simulink subsystem "Controller"  (R2024b)
settings: Solver=VariableStepAuto  StartTime=0.0  StopTime=10.0  RelTol=1e-3
undefined symbols (not defined in the file or in its folder): flight_mode, Parameters, References
libraries: sharedtransform x13, eeGeneralControl x10, simulink x5, aerolibutil x2
(part 1 of 3)
settings Model: Creator=thesa  LastModifiedBy=thesa
settings RTWCC: GPUComputeCapability=3.5

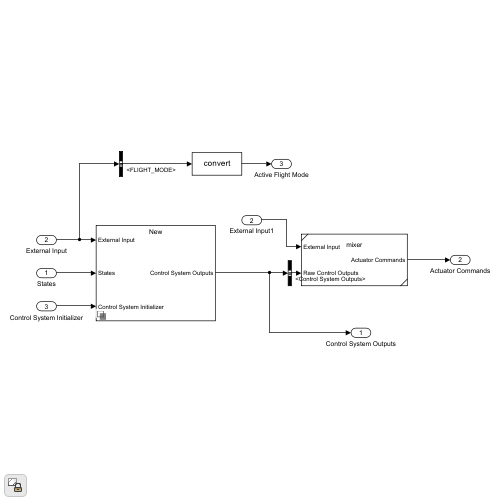
[thumbnail: Simulink's stored preview of the top-level diagram]
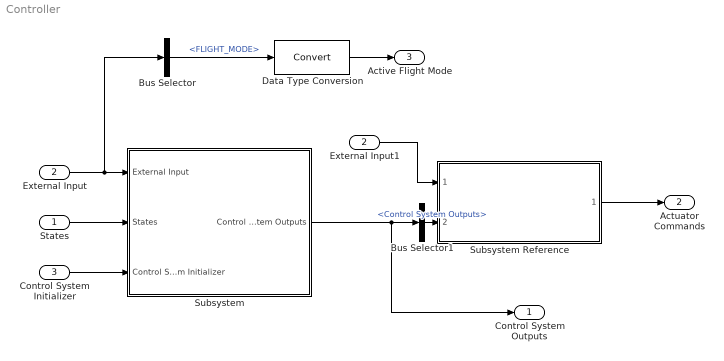
== system Controller ==
  States : Inport
  External Input : Inport  Port=2
  Control System Initializer : Inport  Port=3
  Bus Selector : BusSelector  OutputSignals=Pilot Input.FLIGHT_MODE
  Bus Selector1 : BusSelector  OutputSignals=Control System Outputs
  Data Type Conversion : DataTypeConversion  SaturateOnIntegerOverflow=off  RndMeth=Floor
  External Input1 : InportShadow  Port=2
  Subsystem : Subsystem  Variant=on  VariantControlMode=label  VariantControl=Choice  LabelModeActiveChoice=Choice_1
  Subsystem Reference : Subsystem  ReferencedSubsystem=mixer
  Control System Outputs : Outport
  Actuator Commands : Outport  Port=2
  Active Flight Mode : Outport  Port=3
  wires:
  Control System Initializer/1 -> Subsystem/3(Control System Initializer)
  States/1 -> Subsystem/2(States)
  External Input1/1 -> Subsystem Reference/1
  External Input/1 -> Bus Selector/1, Subsystem/1(External Input)
  Subsystem Reference/1 -> Actuator Commands/1
  Bus Selector/1 -> Data Type Conversion/1  "<FLIGHT_MODE>"
  Subsystem/1(Control System Outputs) -> Bus Selector1/1, Control System Outputs/1
  Data Type Conversion/1 -> Active Flight Mode/1
  Bus Selector1/1 -> Subsystem Reference/2  "<Control System Outputs>"

== system Controller/Subsystem ==
  External Input : Inport
  States : Inport  Port=2
  Control System Initializer : Inport  Port=3
  New : Subsystem  VariantControl=Choice_1
  OLD : Subsystem  VariantControl=Choice
  Control System Outputs : Outport

== system Controller/Subsystem/New ==
  External Input : Inport
  States : Inport  Port=2
  Control System Initializer : Inport  Port=3
  Bus Creator : BusCreator  Inputs=2
  External Input1 : InportShadow
  External Input2 : InportShadow
  Reference Source Selector Logic : Subsystem
  Rotational Motion Feedback Selector : Subsystem
  States2 : InportShadow  Port=2
  States3 : InportShadow  Port=2
  Translational Motion Feedback Selector : Subsystem
  Control System Outputs : Outport
  wires:
  Bus Creator/1 -> Control System Outputs/1
  Translational Motion Feedback Selector/2(Control System Outputs (intermediate)) -> Bus Creator/2  "Control System Outputs (intermediate)"
  Control System Initializer/1 -> Reference Source Selector Logic/3(Initialized Output (in))
  External Input/1 -> Reference Source Selector Logic/2(External Input)
  States/1 -> Reference Source Selector Logic/1(States)
  States3/1 -> Rotational Motion Feedback Selector/3(States)
  External Input2/1 -> Rotational Motion Feedback Selector/2(External Input)
  External Input1/1 -> Translational Motion Feedback Selector/2(External Input)
  States2/1 -> Translational Motion Feedback Selector/3(States)
  Translational Motion Feedback Selector/1(Initialized Output (out)) -> Rotational Motion Feedback Selector/1(Initialized Output (in))
  Rotational Motion Feedback Selector/1(Initialized Output (out)) -> Bus Creator/1  "Control System Outputs"
  Reference Source Selector Logic/1(Initialized Output (out)) -> Translational Motion Feedback Selector/1(Initialized Output (in))

== system Controller/Subsystem/OLD ==
  External Input : Inport
  States : Inport  Port=2
  Control System Initializer : Inport  Port=3
  Bus Selector : BusSelector  OutputSignals=Pilot Input.FLIGHT_MODE
  External Input1 : InportShadow
  Merge : Merge
  Switch Case : SwitchCase  CaseConditions={flight_mode.attitude_control}
  manual control (attitude only) : Subsystem  TreatAsAtomicUnit=on
  position_control + autonomous : Subsystem  TreatAsAtomicUnit=on
  Control System Outputs : Outport
  wires:
  Switch Case/2 -> position_control + autonomous/Action
  Bus Selector/1 -> Switch Case/1  "<FLIGHT_MODE>"
  position_control + autonomous/1(Control System Outputs) -> Merge/2
  States/1 -> manual control (attitude only)/2(States), position_control + autonomous/2(States)
  Switch Case/1 -> manual control (attitude only)/Action
  manual control (attitude only)/1(Control System Outputs) -> Merge/1
  External Input1/1 -> manual control (attitude only)/1(External Input), position_control + autonomous/1(External Input)
  Control System Initializer/1 -> manual control (attitude only)/3(Initialized Output), position_control + autonomous/3(Initialized Output)
  Merge/1 -> Control System Outputs/1
  External Input/1 -> Bus Selector/1

== system Controller/Subsystem/New/Reference Source Selector Logic ==
  States : Inport
  External Input : Inport  Port=2
  Initialized Output (in) : Inport  Port=3
  AUTONOMOUS : Subsystem
  External Input1 : InportShadow  Port=2
  External Input2 : InportShadow  Port=2
  External Input3 : InportShadow  Port=2
  Heading Reference Selection : Subsystem
  States1 : InportShadow
  States2 : InportShadow
  Thrust Reference Selection : Subsystem
  "[X, Y] and/or [Roll, Pitch] Reference Selection" : Subsystem
  Initialized Output (out) : Outport
  wires:
  External Input/1 -> Thrust Reference Selection/2(External Input)
  Initialized Output (in)/1 -> Thrust Reference Selection/1(Initialized Output (in))
  States/1 -> Heading Reference Selection/3(States)
  External Input1/1 -> Heading Reference Selection/2(External Input)
  External Input2/1 -> "[X, Y] and/or [Roll, Pitch] Reference Selection"/2(External Input)
  External Input3/1 -> AUTONOMOUS/2(External Input)
  States1/1 -> "[X, Y] and/or [Roll, Pitch] Reference Selection"/3(States)
  States2/1 -> AUTONOMOUS/3(States)
  AUTONOMOUS/1(Initialized Output (out)) -> Initialized Output (out)/1
  "[X, Y] and/or [Roll, Pitch] Reference Selection"/1(Initialized Output (out)) -> AUTONOMOUS/1(Initialized Output (in))
  Thrust Reference Selection/1(Initialized Output (out)) -> Heading Reference Selection/1(Initialized Output (in))
  Heading Reference Selection/1(Initialized Output (out)) -> "[X, Y] and/or [Roll, Pitch] Reference Selection"/1(Initialized Output (in))

== system Controller/Subsystem/New/Rotational Motion Feedback Selector ==
  Initialized Output (in) : Inport
  External Input : Inport  Port=2
  States : Inport  Port=3
  Bus Creator : BusCreator  Inputs=3
  Bus Selector1 : BusSelector  OutputSignals=External Input.Pilot Input.FLIGHT_MODE
  Merge : Merge
  Pass Through : Subsystem  TreatAsAtomicUnit=on
  Rate Transition : RateTransition  Commented=on  OutPortSampleTime=Parameters.Update_step_s.attitude
  Rate Transition1 : RateTransition  Commented=on
  Switch Case : SwitchCase  CaseConditions={[flight_mode.position_control, flight_mode.position_hold, flight_mode.autonomous, flight_mode.calibration, flight_mode.attitude_control]}
  Switch Case Action Subsystem : Subsystem  TreatAsAtomicUnit=on
  Initialized Output (out) : Outport
  wires:
  Bus Selector1/1 -> Switch Case/1  "<FLIGHT_MODE>"
  Switch Case Action Subsystem/1(Control System Outputs) -> Merge/2
  External Input/1 -> Bus Creator/2  "External Input"
  Pass Through/1(Control System Outputs) -> Merge/1
  Switch Case/2 -> Pass Through/Action
  Switch Case/1 -> Switch Case Action Subsystem/Action
  States/1 -> Bus Creator/3
  Initialized Output (in)/1 -> Bus Creator/1  "Control System Initializer"
  Merge/1 -> Initialized Output (out)/1
  Bus Creator/1 -> Pass Through/1(Combined Control Inputs), Switch Case Action Subsystem/1(Combined Control Inputs), Bus Selector1/1

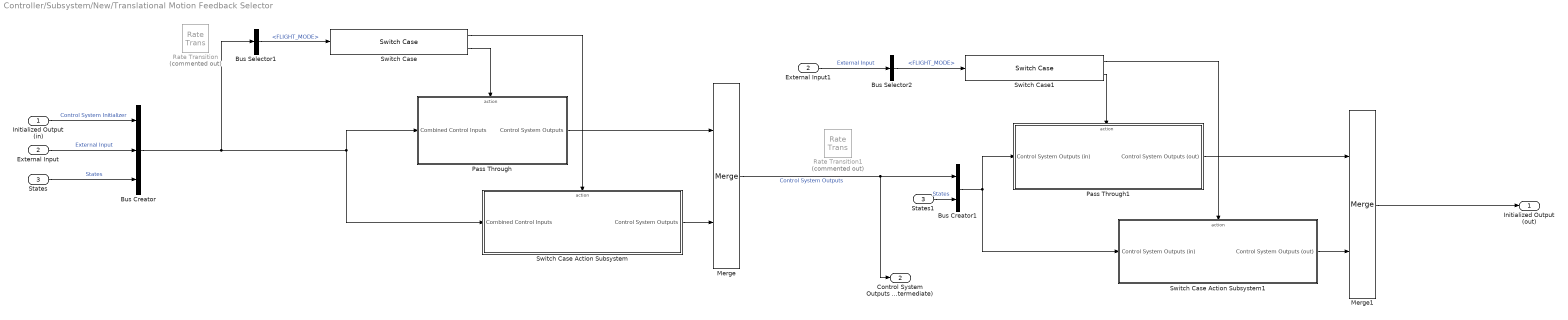
== system Controller/Subsystem/New/Translational Motion Feedback Selector ==
  Initialized Output (in) : Inport
  External Input : Inport  Port=2
  States : Inport  Port=3
  Bus Creator : BusCreator  Inputs=3
  Bus Creator1 : BusCreator  Inputs=2
  Bus Selector1 : BusSelector  OutputSignals=External Input.Pilot Input.FLIGHT_MODE
  Bus Selector2 : BusSelector  OutputSignals=Pilot Input.FLIGHT_MODE
  External Input1 : InportShadow  Port=2
  Merge : Merge
  Merge1 : Merge
  Pass Through : Subsystem  TreatAsAtomicUnit=on
  Pass Through1 : Subsystem  TreatAsAtomicUnit=on
  Rate Transition : RateTransition  Commented=on  OutPortSampleTime=Parameters.Update_step_s.position
  Rate Transition1 : RateTransition  Commented=on  Integrity=off  Deterministic=off
  States1 : InportShadow  Port=3
  Switch Case : SwitchCase  CaseConditions={[flight_mode.position_control, flight_mode.position_hold, flight_mode.autonomous]}
  Switch Case Action Subsystem : Subsystem  TreatAsAtomicUnit=on
  Switch Case Action Subsystem1 : Subsystem  TreatAsAtomicUnit=on
  Switch Case1 : SwitchCase  CaseConditions={[flight_mode.position_control, flight_mode.position_hold, flight_mode.autonomous]}
  Initialized Output (out) : Outport
  Control System Outputs (intermediate) : Outport  Port=2
  wires:
  Bus Selector1/1 -> Switch Case/1  "<FLIGHT_MODE>"
  Switch Case Action Subsystem/1(Control System Outputs) -> Merge/2
  Pass Through/1(Control System Outputs) -> Merge/1
  Switch Case/2 -> Pass Through/Action
  Switch Case/1 -> Switch Case Action Subsystem/Action
  Initialized Output (in)/1 -> Bus Creator/1  "Control System Initializer"
  States/1 -> Bus Creator/3  "States"
  External Input/1 -> Bus Creator/2  "External Input"
  Pass Through1/1(Control System Outputs (out)) -> Merge1/1
  Switch Case1/2 -> Pass Through1/Action
  Bus Creator1/1 -> Pass Through1/1(Control System Outputs (in)), Switch Case Action Subsystem1/1(Control System Outputs (in))
  Switch Case Action Subsystem1/1(Control System Outputs (out)) -> Merge1/2
  Bus Selector2/1 -> Switch Case1/1  "<FLIGHT_MODE>"
  Switch Case1/1 -> Switch Case Action Subsystem1/Action
  External Input1/1 -> Bus Selector2/1  "External Input"
  States1/1 -> Bus Creator1/2  "States"
  Merge1/1 -> Initialized Output (out)/1
  Merge/1 -> Bus Creator1/1, Control System Outputs (intermediate)/1  "Control System Outputs"
  Bus Creator/1 -> Bus Selector1/1, Pass Through/1(Combined Control Inputs), Switch Case Action Subsystem/1(Combined Control Inputs)

== system Controller/Subsystem/OLD/manual control (attitude only) ==
  External Input : Inport
  States : Inport  Port=2
  Initialized Output : Inport  Port=3
  Action Port : ActionPort  InitializeStates=reset
  Subsystem : Subsystem
  Control System Outputs : Outport
  wires:
  Initialized Output/1 -> Subsystem/3(Initialized Output)
  States/1 -> Subsystem/2(States)
  External Input/1 -> Subsystem/1(External Input)
  Subsystem/1(Control Outputs) -> Control System Outputs/1

== system Controller/Subsystem/OLD/position_control + autonomous ==
  External Input : Inport
  States : Inport  Port=2
  Initialized Output : Inport  Port=3
  Action Port : ActionPort  InitializeStates=reset
  Bus Selector : BusSelector  OutputSignals=Control Gains.K_matrix_control.EN
  Guidance : Subsystem
  If : If  IfExpression=u1
  If Action Subsystem : Subsystem  TreatAsAtomicUnit=on
  K-matrix control : Subsystem  TreatAsAtomicUnit=on
  Merge : Merge
  Control System Outputs : Outport
  wires:
  Initialized Output/1 -> Guidance/3(Initialized Output)
  Merge/1 -> Control System Outputs/1
  External Input/1 -> Bus Selector/1, K-matrix control/2(External Inputs), If Action Subsystem/2(External Inputs), Guidance/1(external_input)
  States/1 -> If Action Subsystem/3(States), K-matrix control/3(States), Guidance/2(States)
  Guidance/1(Initialized Output (with references)) -> If Action Subsystem/1(Initialized Output (with references)), K-matrix control/1(Initialized Output (with references))
  If/2 -> If Action Subsystem/Action
  If Action Subsystem/1(Control System Outputs) -> Merge/2
  If/1 -> K-matrix control/Action
  K-matrix control/1(Control System Outputs) -> Merge/1
  Bus Selector/1 -> If/1  "<EN>"

== system Controller/Subsystem/New/Reference Source Selector Logic/AUTONOMOUS ==
  Initialized Output (in) : Inport
  External Input : Inport  Port=2
  States : Inport  Port=3
  Bus Selector : BusSelector  OutputSignals=Pilot Input.FLIGHT_MODE
  External Input1 : InportShadow  Port=2
  Initialized Output (in)1 : InportShadow
  Merge : Merge
  Pass Through : Subsystem  TreatAsAtomicUnit=on
  Switch Case : SwitchCase  CaseConditions={flight_mode.autonomous}
  Use minimum-snap trajectory solution : Subsystem  TreatAsAtomicUnit=on
  Initialized Output (out) : Outport
  wires:
  Initialized Output (in)/1 -> Use minimum-snap trajectory solution/3(Initialized Output)
  States/1 -> Use minimum-snap trajectory solution/2(States)
  Switch Case/1 -> Use minimum-snap trajectory solution/Action
  Bus Selector/1 -> Switch Case/1  "<FLIGHT_MODE>"
  Merge/1 -> Initialized Output (out)/1
  External Input/1 -> Bus Selector/1
  Initialized Output (in)1/1 -> Pass Through/1(Initialized Output (in))
  Use minimum-snap trajectory solution/1(Modified-Initialized Output) -> Merge/2
  External Input1/1 -> Use minimum-snap trajectory solution/1(External Input)
  Switch Case/2 -> Pass Through/Action
  Pass Through/1(Initialized Output (out)) -> Merge/1

== system Controller/Subsystem/New/Reference Source Selector Logic/Heading Reference Selection ==
  Initialized Output (in) : Inport
  External Input : Inport  Port=2
  States : Inport  Port=3
  Bus Selector : BusSelector  OutputSignals=Pilot Input.FLIGHT_MODE
  Direct Yaw Command : Subsystem  TreatAsAtomicUnit=on
  External Input1 : InportShadow  Port=2
  Initialized Output (in)1 : InportShadow
  Merge : Merge
  Pass Through : Subsystem  TreatAsAtomicUnit=on
  Switch Case : SwitchCase  CaseConditions={[flight_mode.position_control, flight_mode.position_hold, flight_mode.calibration, flight_mode.attitude_control]}
  Initialized Output (out) : Outport
  wires:
  Initialized Output (in)1/1 -> Direct Yaw Command/1(Initialized Output (in))
  Merge/1 -> Initialized Output (out)/1
  Switch Case/2 -> Pass Through/Action
  Switch Case/1 -> Direct Yaw Command/Action
  Pass Through/1(Initialized Output (out)) -> Merge/1
  Initialized Output (in)/1 -> Pass Through/1(Initialized Output (in))
  Direct Yaw Command/1(Initialized Output (out)) -> Merge/2
  States/1 -> Direct Yaw Command/3(States)
  Bus Selector/1 -> Switch Case/1  "<FLIGHT_MODE>"
  External Input1/1 -> Direct Yaw Command/2(External Input)
  External Input/1 -> Bus Selector/1

== system Controller/Subsystem/New/Reference Source Selector Logic/Thrust Reference Selection ==
  Initialized Output (in) : Inport
  External Input : Inport  Port=2
  Bus Selector : BusSelector  OutputSignals=Pilot Input.FLIGHT_MODE
  Direct Thrust Command : Subsystem  TreatAsAtomicUnit=on
  Direct Z Position Command : Subsystem  TreatAsAtomicUnit=on
  External Input1 : InportShadow  Port=2
  External Input2 : InportShadow  Port=2
  Initialized Output (in)1 : InportShadow
  Initialized Output (in)2 : InportShadow
  Merge : Merge  Inputs=3
  Pass Through : Subsystem  TreatAsAtomicUnit=on
  Switch Case : SwitchCase  CaseConditions={[flight_mode.position_control, flight_mode.position_hold], [flight_mode.calibration, flight_mode.attitude_control]}
  Initialized Output (out) : Outport
  wires:
  Switch Case/1 -> Direct Z Position Command/Action
  Switch Case/3 -> Pass Through/Action
  Bus Selector/1 -> Switch Case/1  "<FLIGHT_MODE>"
  Switch Case/2 -> Direct Thrust Command/Action
  Pass Through/1(Initialized Output (out)) -> Merge/1
  Direct Z Position Command/1(Initialized Output (out)) -> Merge/3
  Direct Thrust Command/1(Initialized Output (out)) -> Merge/2
  Merge/1 -> Initialized Output (out)/1
  Initialized Output (in)/1 -> Pass Through/1(Initialized Output (in))
  Initialized Output (in)1/1 -> Direct Thrust Command/1(Initialized Output (in))
  Initialized Output (in)2/1 -> Direct Z Position Command/1(Initialized Output (in))
  External Input/1 -> Bus Selector/1
  External Input1/1 -> Direct Z Position Command/2(External Input)
  External Input2/1 -> Direct Thrust Command/2(External Input)

== system Controller/Subsystem/New/Reference Source Selector Logic/[X, Y] and//or [Roll, Pitch] Reference Selection ==
  Initialized Output (in) : Inport
  External Input : Inport  Port=2
  States : Inport  Port=3
  Bus Selector : BusSelector  OutputSignals=Pilot Input.FLIGHT_MODE
  Direct Roll and Pitch Command : Subsystem  TreatAsAtomicUnit=on
  "Direct XY Position Command " : Subsystem  TreatAsAtomicUnit=on
  External Input1 : InportShadow  Port=2
  External Input2 : InportShadow  Port=2
  Initialized Output (in)1 : InportShadow
  Initialized Output (in)2 : InportShadow
  Merge : Merge  Inputs=3
  Pass Through : Subsystem  TreatAsAtomicUnit=on
  Switch Case : SwitchCase  CaseConditions={[flight_mode.position_control, flight_mode.position_hold], [flight_mode.calibration, flight_mode.attitude_control]}
  Initialized Output (out) : Outport
  wires:
  Initialized Output (in)1/1 -> Direct Roll and Pitch Command/1(Initialized Output (in))
  Merge/1 -> Initialized Output (out)/1
  Switch Case/3 -> Pass Through/Action
  Switch Case/2 -> Direct Roll and Pitch Command/Action
  Pass Through/1(Initialized Output (out)) -> Merge/1
  Initialized Output (in)/1 -> Pass Through/1(Initialized Output (in))
  Direct Roll and Pitch Command/1(Initialized Output (out)) -> Merge/2
  States/1 -> "Direct XY Position Command "/3(States)
  External Input1/1 -> Direct Roll and Pitch Command/2(External Input)
  Switch Case/1 -> "Direct XY Position Command "/Action
  "Direct XY Position Command "/1(Initialized Output (out)) -> Merge/3
  Initialized Output (in)2/1 -> "Direct XY Position Command "/1(Initialized Output (in))
  External Input2/1 -> "Direct XY Position Command "/2(External Input)
  External Input/1 -> Bus Selector/1
  Bus Selector/1 -> Switch Case/1  "<FLIGHT_MODE>"

== system Controller/Subsystem/New/Rotational Motion Feedback Selector/Pass Through ==
  Combined Control Inputs : Inport
  Action Port : ActionPort  InitializeStates=reset
  Bus Selector : BusSelector  OutputSignals=Control System Initializer
  Control System Outputs : Outport
  wires:
  Bus Selector/1 -> Control System Outputs/1  "<Control System Initializer>"
  Combined Control Inputs/1 -> Bus Selector/1

== system Controller/Subsystem/New/Rotational Motion Feedback Selector/Switch Case Action Subsystem ==
  Combined Control Inputs : Inport
  Action Port : ActionPort  InitializeStates=reset
  Add : Sum  Inputs=++|
  Attitude Control : Subsystem  ReferencedSubsystem=Attitude_Control
  Bus Assignment : BusAssignment  AssignedSignals=Control Outputs.Tau
  Bus Selector : BusSelector  OutputSignals=Control System Initializer.References.reconstructed.q,Control System Initializer.References.reconstructed.omega,Control System Initializer.References.reconstructed.omega_dot,States,External Input
  Bus Selector1 : BusSelector  OutputSignals=Control System Initializer,Control System Initializer.References.reconstructed.Tau
  Combined Control Inputs1 : InportShadow
  Terminator : Terminator
  Control System Outputs : Outport
  wires:
  Bus Selector/1 -> Attitude Control/1  "<q>"
  Bus Selector/2 -> Attitude Control/2  "<omega>"
  Bus Selector/3 -> Attitude Control/3  "<omega_dot>"
  Bus Selector/4 -> Attitude Control/4  "<States>"
  Bus Selector/5 -> Attitude Control/5  "<External Input>"
  Bus Selector1/2 -> Add/1  "<Tau>"
  Add/1 -> Bus Assignment/2
  Combined Control Inputs/1 -> Bus Selector/1
  Bus Assignment/1 -> Control System Outputs/1
  Combined Control Inputs1/1 -> Bus Selector1/1
  Attitude Control/1 -> Add/2
  Bus Selector1/1 -> Bus Assignment/1  "<Control System Initializer>"
  Attitude Control/2 -> Terminator/1

== system Controller/Subsystem/New/Translational Motion Feedback Selector/Pass Through ==
  Combined Control Inputs : Inport
  Action Port : ActionPort  InitializeStates=reset
  Bus Creator : BusCreator  Inputs=2
  Bus Selector : BusSelector  OutputSignals=Control System Initializer
  Constant : Constant  Value=zeros(3,1)
  Reshape : Reshape
  Control System Outputs : Outport
  wires:
  Bus Selector/1 -> Bus Creator/1  "<Control System Initializer>"
  Combined Control Inputs/1 -> Bus Selector/1
  Bus Creator/1 -> Control System Outputs/1  "Control System Outputs"
  Constant/1 -> Reshape/1
  Reshape/1 -> Bus Creator/2  "thrust_ref"

== system Controller/Subsystem/New/Translational Motion Feedback Selector/Pass Through1 ==
  Control System Outputs (in) : Inport
  Action Port : ActionPort  InitializeStates=reset
  Bus Selector : BusSelector  OutputSignals=Control System Outputs.Control System Initializer
  Control System Outputs (out) : Outport
  wires:
  Bus Selector/1 -> Control System Outputs (out)/1  "<Control System Initializer>"
  Control System Outputs (in)/1 -> Bus Selector/1

== system Controller/Subsystem/New/Translational Motion Feedback Selector/Switch Case Action Subsystem ==
  Combined Control Inputs : Inport
  Action Port : ActionPort  InitializeStates=reset
  Bus Selector : BusSelector  OutputSignals=Control System Initializer,External Input,States
  Translational Motion Control : Subsystem  VariantControl=Choice_1
  Control System Outputs : Outport
  wires:
  Bus Selector/2 -> Translational Motion Control/2(External Inputs)  "<External Input>"
  Combined Control Inputs/1 -> Bus Selector/1
  Bus Selector/3 -> Translational Motion Control/3(States)  "<States>"
  Bus Selector/1 -> Translational Motion Control/1(Initialized Output (with references))  "<Control System Initializer>"
  Translational Motion Control/1(Control System Outputs) -> Control System Outputs/1

== system Controller/Subsystem/New/Translational Motion Feedback Selector/Switch Case Action Subsystem1 ==
  Control System Outputs (in) : Inport
  Action Port : ActionPort  InitializeStates=reset
  Bus Selector : BusSelector  OutputSignals=Control System Outputs.thrust_ref,Control System Outputs
  Translational Motion Control : Subsystem  VariantControl=Choice_1
  Control System Outputs (out) : Outport
  wires:
  Control System Outputs (in)/1 -> Bus Selector/1
  Bus Selector/2 -> Translational Motion Control/2(Control System Outputs (in))  "<Control System Outputs>"
  Translational Motion Control/1(Control System Outputs (out)) -> Control System Outputs (out)/1
  Bus Selector/1 -> Translational Motion Control/1(thrust_ref)  "<thrust_ref>"

== system Controller/Subsystem/OLD/manual control (attitude only)/Subsystem ==
  External Input : Inport
  States : Inport  Port=2
  Initialized Output : Inport  Port=3
  External Input1 : InportShadow
  Map User Input : Subsystem
  Reshape2 : Reshape  OutputDimensionality=Column vector (2-D)
  States1 : InportShadow  Port=2
  Subsystem : Subsystem
  Subsystem1 : Subsystem
  Subsystem2 : Subsystem  Commented=on
  Control Outputs : Outport
  wires:
  Initialized Output/1 -> Subsystem1/6(Initialized Output)
  States/1 -> Map User Input/2(States)
  Subsystem1/1(Control Outputs) -> Control Outputs/1
  External Input/1 -> Map User Input/1(External Input)
  Map User Input/2(att_ref) -> Subsystem/1(att_ref), Subsystem1/2(att_ref)
  Reshape2/1 -> Subsystem/2(omega_ref), Subsystem1/3(omega_ref)
  Map User Input/1(T_ref) -> Subsystem1/1(T)  "T"
  Map User Input/3(omega_ref) -> Reshape2/1
  Map User Input/4(omega_dot_ref) -> Subsystem/3(omega_dot_ref)
  External Input1/1 -> Subsystem/5(External Input)
  States1/1 -> Subsystem/4(States)
  Subsystem/2(Tau) -> Subsystem1/5(Tau)
  Subsystem/1(omega_dot) -> Subsystem1/4(omega_dot)

== system Controller/Subsystem/OLD/position_control + autonomous/Guidance ==
  external_input : Inport
  States : Inport  Port=2
  Initialized Output : Inport  Port=3
  Trajectory Solution Evaluator : Subsystem
  Initialized Output (with references) : Outport
  wires:
  Initialized Output/1 -> Trajectory Solution Evaluator/3(Initialized Output)
  States/1 -> Trajectory Solution Evaluator/2(States)
  Trajectory Solution Evaluator/1(Initialized Output (with references)) -> Initialized Output (with references)/1
  external_input/1 -> Trajectory Solution Evaluator/1(external_input)

== system Controller/Subsystem/OLD/position_control + autonomous/If Action Subsystem ==
  Initialized Output (with references) : Inport
  External Inputs : Inport  Port=2
  States : Inport  Port=3
  Action Port : ActionPort
  Attitude + Position FF control : Subsystem  Commented=on  VariantControl=Choice_1
  Attitude + Position FF control1 : Subsystem  Commented=on  VariantControl=Choice_1
  Attitude + Position FF control2 : Subsystem  VariantControl=Choice_1
  Control System Outputs : Outport
  wires:
  States/1 -> Attitude + Position FF control2/3(States)
  External Inputs/1 -> Attitude + Position FF control2/2(External Inputs)
  Initialized Output (with references)/1 -> Attitude + Position FF control2/1(Initialized Output (with references))
  Attitude + Position FF control2/1(Control System Outputs) -> Control System Outputs/1

== system Controller/Subsystem/OLD/position_control + autonomous/K-matrix control ==
  Initialized Output (with references) : Inport
  External Inputs : Inport  Port=2
  States : Inport  Port=3
  Action Port : ActionPort
  K-matrix-control : Subsystem  VariantControl=Choice
  Control System Outputs : Outport
  wires:
  States/1 -> K-matrix-control/3(States)
  External Inputs/1 -> K-matrix-control/2(External Inputs)
  Initialized Output (with references)/1 -> K-matrix-control/1(Initialized Output (with references))
  K-matrix-control/1(Control System Outputs) -> Control System Outputs/1

== system Controller/Subsystem/New/Reference Source Selector Logic/AUTONOMOUS/Pass Through ==
  Initialized Output (in) : Inport
  Action Port : ActionPort  InitializeStates=reset
  Initialized Output (out) : Outport
  wires:
  Initialized Output (in)/1 -> Initialized Output (out)/1

== system Controller/Subsystem/New/Reference Source Selector Logic/AUTONOMOUS/Use minimum-snap trajectory solution ==
  External Input : Inport
  States : Inport  Port=2
  Initialized Output : Inport  Port=3
  Action Port : ActionPort  InitializeStates=reset
  FF reconstructor : Subsystem  ReferencedSubsystem=FF_reconstructor
  Modified-Initialized Output : Outport
  wires:
  External Input/1 -> FF reconstructor/2
  States/1 -> FF reconstructor/3
  FF reconstructor/1 -> Modified-Initialized Output/1
  Initialized Output/1 -> FF reconstructor/1

== system Controller/Subsystem/New/Reference Source Selector Logic/Heading Reference Selection/Direct Yaw Command ==
  Initialized Output (in) : Inport
  External Input : Inport  Port=2
  States : Inport  Port=3
  Action Port : ActionPort  InitializeStates=reset
  Direct Yaw Command : Subsystem  ReferencedSubsystem=Direct_Yaw_Command
  Subsystem : Subsystem
  Initialized Output (out) : Outport
  wires:
  External Input/1 -> Direct Yaw Command/1
  Initialized Output (in)/1 -> Subsystem/4(Initialized Output)
  Subsystem/1(Modified-Initialized Output) -> Initialized Output (out)/1
  States/1 -> Direct Yaw Command/2
  Direct Yaw Command/3 -> Subsystem/3(yaw_acc_ref)
  Direct Yaw Command/2 -> Subsystem/2(yaw_rate_ref)
  Direct Yaw Command/1 -> Subsystem/1(yaw_ref)

== system Controller/Subsystem/New/Reference Source Selector Logic/Heading Reference Selection/Pass Through ==
  Initialized Output (in) : Inport
  Action Port : ActionPort  InitializeStates=reset
  Initialized Output (out) : Outport
  wires:
  Initialized Output (in)/1 -> Initialized Output (out)/1

== system Controller/Subsystem/New/Reference Source Selector Logic/Thrust Reference Selection/Direct Thrust Command ==
  Initialized Output (in) : Inport
  External Input : Inport  Port=2
  Action Port : ActionPort  InitializeStates=reset
  Direct Thrust Command : Subsystem  ReferencedSubsystem=Direct_Thrust_Command
  Subsystem1 : Subsystem
  Initialized Output (out) : Outport
  wires:
  External Input/1 -> Direct Thrust Command/1
  Initialized Output (in)/1 -> Subsystem1/2(Initialized Output)
  Subsystem1/1(Control Outputs) -> Initialized Output (out)/1
  Direct Thrust Command/1 -> Subsystem1/1(T)

== system Controller/Subsystem/New/Reference Source Selector Logic/Thrust Reference Selection/Direct Z Position Command ==
  Initialized Output (in) : Inport
  External Input : Inport  Port=2
  Action Port : ActionPort  InitializeStates=reset
  Direct Z Position Command : Subsystem  ReferencedSubsystem=Direct_Z_Position_Command
  Initialized Output (in)1 : InportShadow
  Subsystem : Subsystem
  Initialized Output (out) : Outport
  wires:
  External Input/1 -> Direct Z Position Command/1
  Initialized Output (in)/1 -> Subsystem/4(Initialized Output)
  Subsystem/1(Modified-Initialized Output) -> Initialized Output (out)/1
  Initialized Output (in)1/1 -> Direct Z Position Command/2
  Direct Z Position Command/1 -> Subsystem/1(Z_e_ref)
  Direct Z Position Command/2 -> Subsystem/2(Vz_e_ref)
  Direct Z Position Command/3 -> Subsystem/3(Az_e_ref)

== system Controller/Subsystem/New/Reference Source Selector Logic/Thrust Reference Selection/Pass Through ==
  Initialized Output (in) : Inport
  Action Port : ActionPort  InitializeStates=reset
  Initialized Output (out) : Outport
  wires:
  Initialized Output (in)/1 -> Initialized Output (out)/1

== system Controller/Subsystem/New/Reference Source Selector Logic/[X, Y] and//or [Roll, Pitch] Reference Selection/Direct Roll and Pitch Command ==
  Initialized Output (in) : Inport
  External Input : Inport  Port=2
  Action Port : ActionPort  InitializeStates=reset
  Direct Roll and Pitch Command : Subsystem  ReferencedSubsystem=Direct_Roll_and_Pitch_Command
  Subsystem1 : Subsystem
  Initialized Output (out) : Outport
  wires:
  External Input/1 -> Direct Roll and Pitch Command/1
  Initialized Output (in)/1 -> Subsystem1/4(Initialized Output)
  Subsystem1/1(Control Outputs) -> Initialized Output (out)/1
  Direct Roll and Pitch Command/1 -> Subsystem1/1(Roll_Pitch_ref)
  Direct Roll and Pitch Command/2 -> Subsystem1/2(Roll_Pitch_Rate_ref)
  Direct Roll and Pitch Command/3 -> Subsystem1/3(Roll_Pitch_Acc_ref)

== system Controller/Subsystem/New/Reference Source Selector Logic/[X, Y] and//or [Roll, Pitch] Reference Selection/Direct XY Position Command  ==
  Initialized Output (in) : Inport
  External Input : Inport  Port=2
  States : Inport  Port=3
  Action Port : ActionPort  InitializeStates=reset
  "Direct XY Position Command " : Subsystem
  Initialized Output (in)1 : InportShadow
  Subsystem1 : Subsystem
  Initialized Output (out) : Outport
  wires:
  External Input/1 -> "Direct XY Position Command "/1(External Input)
  Initialized Output (in)/1 -> Subsystem1/4(Initialized Output)
  Subsystem1/1(Control Outputs) -> Initialized Output (out)/1
  "Direct XY Position Command "/1(XY_e_ref) -> Subsystem1/1(XY_e_ref)
  "Direct XY Position Command "/2(Vxy_e_ref) -> Subsystem1/2(Vxy_e_ref)
  "Direct XY Position Command "/3(Axy_e_ref) -> Subsystem1/3(Axy_e_ref)
  States/1 -> "Direct XY Position Command "/2(States)
  Initialized Output (in)1/1 -> "Direct XY Position Command "/3(Initialized Output)

== system Controller/Subsystem/New/Reference Source Selector Logic/[X, Y] and//or [Roll, Pitch] Reference Selection/Pass Through ==
  Initialized Output (in) : Inport
  Action Port : ActionPort  InitializeStates=reset
  Initialized Output (out) : Outport
  wires:
  Initialized Output (in)/1 -> Initialized Output (out)/1

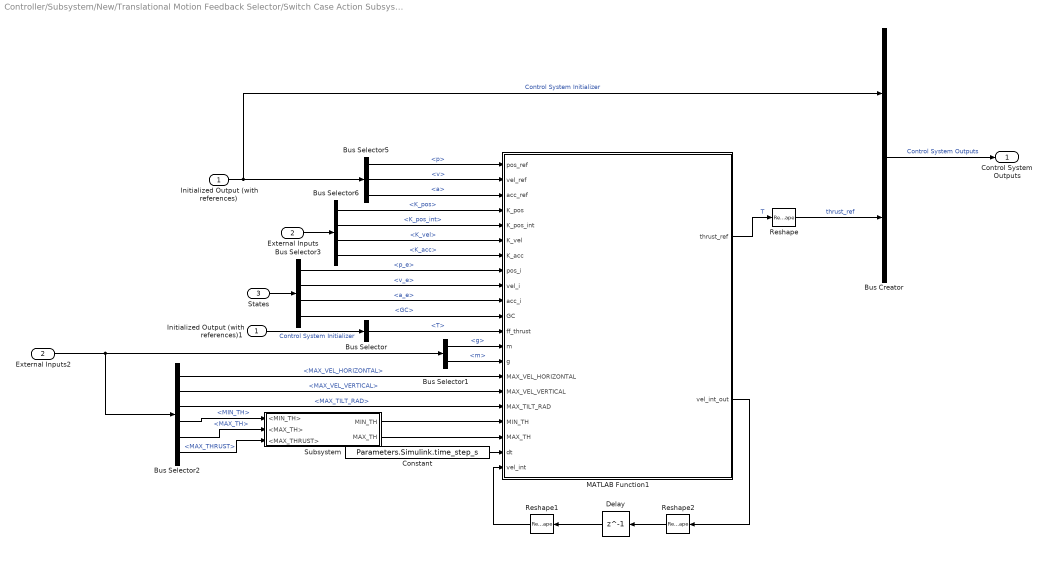
== system Controller/Subsystem/New/Translational Motion Feedback Selector/Switch Case Action Subsystem/Translational Motion Control ==
  Initialized Output (with references) : Inport
  External Inputs : Inport  Port=2
  States : Inport  Port=3
  Bus Creator : BusCreator  Inputs=2
  Bus Selector : BusSelector  OutputSignals=References.reconstructed.T
  Bus Selector1 : BusSelector  OutputSignals=Vehicle Parameters.g,Vehicle Parameters.m
  Bus Selector2 : BusSelector  OutputSignals=Control Logic.MAX_VEL_HORIZONTAL,Control Logic.MAX_VEL_VERTICAL,Control Logic.MAX_TILT_RAD,Control Logic.MIN_TH,Control Logic.MAX_TH,Vehicle Parameters.MAX_THRUST
  Bus Selector3 : BusSelector  OutputSignals=p_e,v_e,a_e,GC
  Bus Selector5 : BusSelector  OutputSignals=References.trajectory.p,References.trajectory.v,References.trajectory.a
  Bus Selector6 : BusSelector  OutputSignals=Control Gains.K_pos,Control Gains.K_pos_int,Control Gains.K_vel,Control Gains.K_acc
  Constant : Constant  Value=Parameters.Simulink.time_step_s
  Delay : Delay  DelayLength=1  InitialCondition=zeros(3,1)
  External Inputs2 : InportShadow  Port=2
  Initialized Output (with references)1 : InportShadow
  MATLAB Function1 : MATLAB Function  TreatAsAtomicUnit=on
  Reshape : Reshape
  Reshape1 : Reshape  OutputDimensionality=Column vector (2-D)
  Reshape2 : Reshape  OutputDimensionality=Column vector (2-D)
  Subsystem : Subsystem
  Control System Outputs : Outport
  wires:
  Bus Selector6/2 -> MATLAB Function1/5(K_pos_int)  "<K_pos_int>"
  Bus Selector6/4 -> MATLAB Function1/7(K_acc)  "<K_acc>"
  Bus Selector6/3 -> MATLAB Function1/6(K_vel)  "<K_vel>"
  Bus Selector6/1 -> MATLAB Function1/4(K_pos)  "<K_pos>"
  Bus Selector3/3 -> MATLAB Function1/10(acc_i)  "<a_e>"
  Bus Selector3/2 -> MATLAB Function1/9(vel_i)  "<v_e>"
  Bus Selector3/1 -> MATLAB Function1/8(pos_i)  "<p_e>"
  Bus Selector5/3 -> MATLAB Function1/3(acc_ref)  "<a>"
  Bus Selector5/2 -> MATLAB Function1/2(vel_ref)  "<v>"
  Bus Selector5/1 -> MATLAB Function1/1(pos_ref)  "<p>"
  Initialized Output (with references)/1 -> Bus Creator/1, Bus Selector5/1  "Control System Initializer"
  MATLAB Function1/1(thrust_ref) -> Reshape/1  "T"
  External Inputs/1 -> Bus Selector6/1
  States/1 -> Bus Selector3/1
  Reshape/1 -> Bus Creator/2  "thrust_ref"
  Bus Creator/1 -> Control System Outputs/1  "Control System Outputs"
  MATLAB Function1/2(vel_int_out) -> Reshape2/1
  Delay/1 -> Reshape1/1
  External Inputs2/1 -> Bus Selector1/1, Bus Selector2/1
  Bus Selector1/1 -> MATLAB Function1/13(m)  "<g>"
  Bus Selector1/2 -> MATLAB Function1/14(g)  "<m>"
  Constant/1 -> MATLAB Function1/20(dt)
  Reshape1/1 -> MATLAB Function1/21(vel_int)
  Reshape2/1 -> Delay/1
  Bus Selector3/4 -> MATLAB Function1/11(GC)  "<GC>"
  Initialized Output (with references)1/1 -> Bus Selector/1  "Control System Initializer"
  Bus Selector/1 -> MATLAB Function1/12(ff_thrust)  "<T>"
  Bus Selector2/3 -> MATLAB Function1/17(MAX_TILT_RAD)  "<MAX_TILT_RAD>"
  Bus Selector2/5 -> Subsystem/2(<MAX_TH>)  "<MAX_TH>"
  Bus Selector2/4 -> Subsystem/1(<MIN_TH>)  "<MIN_TH>"
  Subsystem/1(MIN_TH) -> MATLAB Function1/18(MIN_TH)
  Subsystem/2(MAX_TH) -> MATLAB Function1/19(MAX_TH)
  Bus Selector2/6 -> Subsystem/3(<MAX_THRUST>)  "<MAX_THRUST>"
  Bus Selector2/2 -> MATLAB Function1/16(MAX_VEL_VERTICAL)  "<MAX_VEL_VERTICAL>"
  Bus Selector2/1 -> MATLAB Function1/15(MAX_VEL_HORIZONTAL)  "<MAX_VEL_HORIZONTAL>"

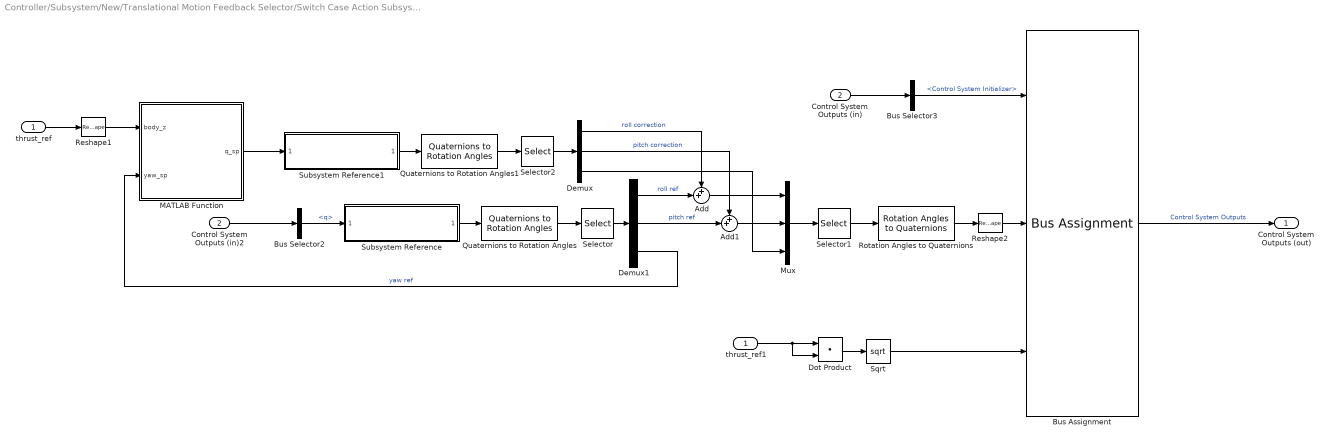
== system Controller/Subsystem/New/Translational Motion Feedback Selector/Switch Case Action Subsystem1/Translational Motion Control ==
  thrust_ref : Inport
  Control System Outputs (in) : Inport  Port=2
  Add : Sum  Inputs=++|
  Add1 : Sum  Inputs=++|
  Bus Assignment : BusAssignment  AssignedSignals=References.reconstructed.q,Control Outputs.T
  Bus Selector2 : BusSelector  OutputSignals=Control System Initializer.References.reconstructed.q
  Bus Selector3 : BusSelector  OutputSignals=Control System Initializer
  Control System Outputs (in)2 : InportShadow  Port=2
  Demux : Demux  Outputs=3
  Demux1 : Demux  Outputs=3
  Dot Product : DotProduct  OutDataTypeStr=Inherit: Inherit via internal rule
  MATLAB Function : MATLAB Function  TreatAsAtomicUnit=on
  Mux : Mux  Inputs=3
  Quaternions to Rotation Angles : sharedtransform/Quaternions to Rotation Angles  rotationOrder=ZYX  aMode=aMode
  Quaternions to Rotation Angles1 : sharedtransform/Quaternions to Rotation Angles  rotationOrder=ZYX  aMode=aMode
  Reshape1 : Reshape  OutputDimensionality=Column vector (2-D)
  Reshape2 : Reshape  OutputDimensionality=Row vector (2-D)
  Rotation Angles to Quaternions : sharedtransform/Rotation Angles to Quaternions  rotationOrder=ZYX  aMode=aMode
  Selector : Selector  InputPortWidth=3  IndexOptions=Index vector (dialog)  Indices=[3 2 1]  OutputSizes=1
  Selector1 : Selector  InputPortWidth=3  IndexOptions=Index vector (dialog)  Indices=[3 2 1]  OutputSizes=1
  Selector2 : Selector  InputPortWidth=3  IndexOptions=Index vector (dialog)  Indices=[3 2 1]  OutputSizes=1
  Sqrt : Sqrt
  Subsystem Reference : Subsystem  ReferencedSubsystem=Check_Quat
  Subsystem Reference1 : Subsystem  ReferencedSubsystem=Check_Quat
  thrust_ref1 : InportShadow
  Control System Outputs (out) : Outport
  wires:
  Sqrt/1 -> Bus Assignment/3
  Bus Assignment/1 -> Control System Outputs (out)/1  "Control System Outputs"
  Bus Selector3/1 -> Bus Assignment/1  "<Control System Initializer>"
  Control System Outputs (in)/1 -> Bus Selector3/1
  thrust_ref1/1 -> Dot Product/2, Dot Product/1
  Dot Product/1 -> Sqrt/1
  Demux1/1 -> Add/2  "roll ref"
  Demux1/2 -> Add1/2  "pitch ref"
  Add1/1 -> Mux/2
  Reshape2/1 -> Bus Assignment/2
  Selector1/1 -> Rotation Angles to Quaternions/1
  Demux/2 -> Add1/1  "pitch correction"
  Demux1/3 -> MATLAB Function/2(yaw_sp)  "yaw ref"
  Demux/1 -> Add/1  "roll correction"
  Quaternions to Rotation Angles/1 -> Selector/1
  Add/1 -> Mux/1
  Selector/1 -> Demux1/1
  Mux/1 -> Selector1/1
  Bus Selector2/1 -> Subsystem Reference/1  "<q>"
  Subsystem Reference/1 -> Quaternions to Rotation Angles/1
  Subsystem Reference1/1 -> Quaternions to Rotation Angles1/1
  Selector2/1 -> Demux/1
  Quaternions to Rotation Angles1/1 -> Selector2/1
  Rotation Angles to Quaternions/1 -> Reshape2/1
  MATLAB Function/1(q_sp) -> Subsystem Reference1/1
  Demux/3 -> Mux/3
  Control System Outputs (in)2/1 -> Bus Selector2/1
  thrust_ref/1 -> Reshape1/1
  Reshape1/1 -> MATLAB Function/1(body_z)

== system Controller/Subsystem/OLD/manual control (attitude only)/Subsystem/Map User Input ==
  External Input : Inport
  States : Inport  Port=2
  Direct Roll and Pitch Command : Subsystem  ReferencedSubsystem=Direct_Roll_and_Pitch_Command
  Mux1 : Mux  Inputs=2
  Mux2 : Mux  Inputs=2
  Mux3 : Mux  Inputs=2
  Subsystem Reference : Subsystem  ReferencedSubsystem=Direct_Thrust_Command
  Subsystem Reference1 : Subsystem  ReferencedSubsystem=Direct_Yaw_Command
  T_ref : Outport
  att_ref : Outport  Port=2
  omega_ref : Outport  Port=3
  omega_dot_ref : Outport  Port=4
  wires:
  External Input/1 -> Subsystem Reference1/1, Direct Roll and Pitch Command/1, Subsystem Reference/1
  Mux1/1 -> omega_ref/1
  Subsystem Reference/1 -> T_ref/1
  Mux2/1 -> omega_dot_ref/1
  Direct Roll and Pitch Command/2 -> Mux1/1
  Direct Roll and Pitch Command/3 -> Mux2/1
  Subsystem Reference1/2 -> Mux1/2
  Subsystem Reference1/3 -> Mux2/2
  States/1 -> Subsystem Reference1/2
  Mux3/1 -> att_ref/1
  Subsystem Reference1/1 -> Mux3/2
  Direct Roll and Pitch Command/1 -> Mux3/1

== system Controller/Subsystem/OLD/manual control (attitude only)/Subsystem/Subsystem ==
  att_ref : Inport
  omega_ref : Inport  Port=2
  omega_dot_ref : Inport  Port=3
  States : Inport  Port=4
  External Input : Inport  Port=5
  Attitude Control : Subsystem  ReferencedSubsystem=Attitude_Control
  Reshape : Reshape  OutputDimensionality=Row vector (2-D)
  Rotation Angles to Quaternions : sharedtransform/Rotation Angles to Quaternions  rotationOrder=ZYX  aMode=aMode
  Selector : Selector  InputPortWidth=3  IndexOptions=Index vector (dialog)  Indices=[3 2 1]  OutputSizes=1
  omega_dot : Outport
  Tau : Outport  Port=2
  wires:
  States/1 -> Attitude Control/4
  omega_ref/1 -> Attitude Control/2
  Attitude Control/1 -> Tau/1
  External Input/1 -> Attitude Control/5
  att_ref/1 -> Selector/1
  Attitude Control/2 -> omega_dot/1
  Reshape/1 -> Attitude Control/1
  Rotation Angles to Quaternions/1 -> Reshape/1
  omega_dot_ref/1 -> Attitude Control/3
  Selector/1 -> Rotation Angles to Quaternions/1

== system Controller/Subsystem/OLD/manual control (attitude only)/Subsystem/Subsystem1 ==
  T : Inport
  att_ref : Inport  Port=2
  omega_ref : Inport  Port=3
  omega_dot : Inport  Port=4
  Tau : Inport  Port=5
  Initialized Output : Inport  Port=6
  Bus Assignment : BusAssignment  AssignedSignals=References.trajectory.psi,References.trajectory.psi_dot,References.reconstructed.q,References.reconstructed.omega,References.reconstructed.omega_dot,References.reconstructed.T,Control Outputs.T,References.reconstructed.Tau,Control Outputs.Tau
  Reshape10 : Reshape  OutputDimensionality=Column vector (2-D)
  Reshape11 : Reshape  OutputDimensionality=Row vector (2-D)
  Reshape7 : Reshape  OutputDimensionality=Column vector (2-D)
  Reshape8 : Reshape  OutputDimensionality=Column vector (2-D)
  Rotation Angles to Quaternions : sharedtransform/Rotation Angles to Quaternions  rotationOrder=ZYX  aMode=aMode
  Selector : Selector  InputPortWidth=3  IndexOptions=Index vector (dialog)  Indices=[3]  OutputSizes=1
  Selector1 : Selector  InputPortWidth=3  IndexOptions=Index vector (dialog)  Indices=[3]  OutputSizes=1
  Selector2 : Selector  InputPortWidth=3  IndexOptions=Index vector (dialog)  Indices=[3 2 1]  OutputSizes=1
  Control Outputs : Outport
  wires:
  Selector2/1 -> Rotation Angles to Quaternions/1
  Bus Assignment/1 -> Control Outputs/1
  Initialized Output/1 -> Bus Assignment/1
  Reshape10/1 -> Bus Assignment/10, Bus Assignment/9  "Tau"
  omega_dot/1 -> Reshape8/1
  Reshape11/1 -> Bus Assignment/4  "q"
  Reshape8/1 -> Bus Assignment/6  "omega_dot"
  Rotation Angles to Quaternions/1 -> Reshape11/1  "q"
  Reshape7/1 -> Bus Assignment/5  "omega"
  T/1 -> Bus Assignment/8, Bus Assignment/7  "T"
  att_ref/1 -> Selector2/1, Selector1/1
  omega_ref/1 -> Selector/1, Reshape7/1
  Tau/1 -> Reshape10/1
  Selector/1 -> Bus Assignment/3  "psi_dot"
  Selector1/1 -> Bus Assignment/2  "psi"

== system Controller/Subsystem/OLD/manual control (attitude only)/Subsystem/Subsystem2 ==
  att_ref : Inport
  omega_ref : Inport  Port=2
  States : Inport  Port=3
  External Input : Inport  Port=4
  Add : Sum  Inputs=|++
  Add2 : Sum  Inputs=-+|
  Bus Selector : BusSelector  OutputSignals=q,omega
  Bus Selector4 : BusSelector  OutputSignals=Control Gains.K_att,Vehicle Parameters.J,Control Gains.K_omega
  MATLAB Function2 : MATLAB Function  TreatAsAtomicUnit=on
  Matrix Multiply : Product  Multiplication=Matrix(*)
  Matrix Multiply1 : Product  Multiplication=Matrix(*)
  Matrix Multiply2 : Product  Multiplication=Matrix(*)
  Reshape1 : Reshape  OutputDimensionality=Column vector (2-D)
  Reshape3 : Reshape  OutputDimensionality=Column vector (2-D)
  Reshape4 : Reshape  OutputDimensionality=Column vector (2-D)
  Signed Square Root : Sqrt  Operator=signedSqrt  OutputSignalType=real
  omega_dot : Outport
  Tau : Outport  Port=2
  wires:
  Reshape4/1 -> Add/1
  MATLAB Function2/1(rpy_rate_fb) -> Reshape1/1
  Bus Selector/1 -> MATLAB Function2/1(q)  "<q>"
  Bus Selector4/1 -> Matrix Multiply/1  "<K_att>"
  omega_ref/1 -> Add2/2
  Add/1 -> omega_dot/1, Matrix Multiply2/2
  att_ref/1 -> MATLAB Function2/2(att_ref)
  Bus Selector4/2 -> Matrix Multiply2/1  "<J>"
  Matrix Multiply1/1 -> Add/2
  Matrix Multiply/1 -> Reshape4/1
  Signed Square Root/1 -> Matrix Multiply1/2
  Reshape1/1 -> Matrix Multiply/2
  Add2/1 -> Signed Square Root/1
  Matrix Multiply2/1 -> Tau/1
  Bus Selector/2 -> Reshape3/1  "<omega>"
  Reshape3/1 -> Add2/1
  Bus Selector4/3 -> Matrix Multiply1/1  "<K_omega>"
  External Input/1 -> Bus Selector4/1
  States/1 -> Bus Selector/1

== system Controller/Subsystem/OLD/position_control + autonomous/Guidance/Trajectory Solution Evaluator ==
  external_input : Inport
  States : Inport  Port=2
  Initialized Output : Inport  Port=3
  Bus Selector : BusSelector  OutputSignals=Pilot Input.FLIGHT_MODE
  Hold current position : Subsystem  TreatAsAtomicUnit=on
  Merge : Merge  Inputs=3
  Switch Case : SwitchCase  CaseConditions={flight_mode.autonomous, flight_mode.position_control}
  Switch Case Action Subsystem : Subsystem  TreatAsAtomicUnit=on
  Switch Case Action Subsystem1 : Subsystem  TreatAsAtomicUnit=on
  Initialized Output (with references) : Outport
  wires:
  Switch Case/3 -> Hold current position/Action
  Switch Case/2 -> Switch Case Action Subsystem1/Action
  Switch Case Action Subsystem1/1(Modified-Initialized Output) -> Merge/3
  Initialized Output/1 -> Hold current position/1(Initialized Output), Switch Case Action Subsystem/3(Initialized Output), Switch Case Action Subsystem1/3(Initialized Output)
  States/1 -> Switch Case Action Subsystem/2(States), Switch Case Action Subsystem1/1(States)
  Switch Case/1 -> Switch Case Action Subsystem/Action
  Bus Selector/1 -> Switch Case/1  "<FLIGHT_MODE>"
  Switch Case Action Subsystem/1(Modified-Initialized Output) -> Merge/1
  Merge/1 -> Initialized Output (with references)/1
  Hold current position/1(Modified-Initialized Output) -> Merge/2
  external_input/1 -> Switch Case Action Subsystem/1(external_input), Bus Selector/1, Switch Case Action Subsystem1/2(external_input)

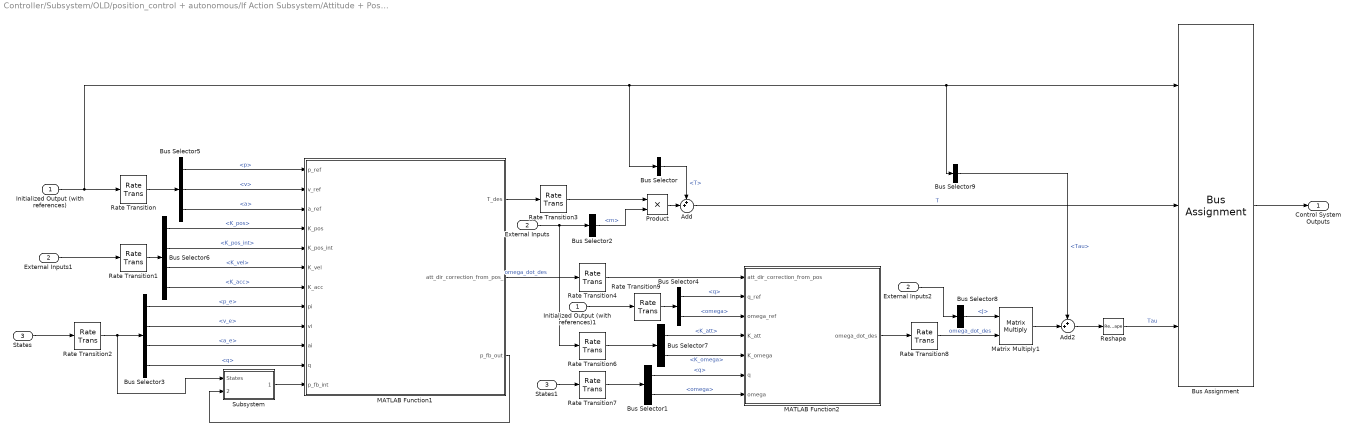
== system Controller/Subsystem/OLD/position_control + autonomous/If Action Subsystem/Attitude + Position FF control ==
  Initialized Output (with references) : Inport
  External Inputs : Inport  Port=2
  States : Inport  Port=3
  Add : Sum  Inputs=++|
  Add2 : Sum  Inputs=++|
  Bus Assignment : BusAssignment  AssignedSignals=Control Outputs.T,Control Outputs.Tau
  Bus Selector : BusSelector  OutputSignals=References.reconstructed.T
  Bus Selector1 : BusSelector  OutputSignals=q,omega
  Bus Selector2 : BusSelector  OutputSignals=Vehicle Parameters.m
  Bus Selector3 : BusSelector  OutputSignals=p_e,v_e,a_e,q
  Bus Selector4 : BusSelector  OutputSignals=References.reconstructed.q,References.reconstructed.omega
  Bus Selector5 : BusSelector  OutputSignals=References.trajectory.p,References.trajectory.v,References.trajectory.a
  Bus Selector6 : BusSelector  OutputSignals=Control Gains.K_pos,Control Gains.K_pos_int,Control Gains.K_vel,Control Gains.K_acc
  Bus Selector7 : BusSelector  OutputSignals=Control Gains.K_att,Control Gains.K_omega
  Bus Selector8 : BusSelector  OutputSignals=Vehicle Parameters.J
  Bus Selector9 : BusSelector  OutputSignals=References.reconstructed.Tau
  External Inputs1 : InportShadow  Port=2
  External Inputs2 : InportShadow  Port=2
  Initialized Output (with references)1 : InportShadow
  MATLAB Function1 : MATLAB Function  TreatAsAtomicUnit=on
  MATLAB Function2 : MATLAB Function  TreatAsAtomicUnit=on
  Matrix Multiply1 : Product  Multiplication=Matrix(*)
  Product : Product
  Rate Transition : RateTransition  OutPortSampleTime=Parameters.Update_step_s.position
  Rate Transition1 : RateTransition  OutPortSampleTime=Parameters.Update_step_s.position
  Rate Transition2 : RateTransition  OutPortSampleTime=Parameters.Update_step_s.position
  Rate Transition3 : RateTransition
  Rate Transition{4,6..7,9} (4 alike) : RateTransition  OutPortSampleTime=Parameters.Update_step_s.attitude
  Rate Transition8 : RateTransition
  Reshape : Reshape  OutputDimensionality=Column vector (2-D)
  States1 : InportShadow  Port=3
  Subsystem : Subsystem
  Control System Outputs : Outport
  wires:
  Bus Selector9/1 -> Add2/1  "<Tau>"
  Subsystem/1(p_fb_int) -> MATLAB Function1/12(p_fb_int)
  MATLAB Function1/3(p_fb_out) -> Subsystem/2(p_fb_out)
  Bus Selector6/2 -> MATLAB Function1/5(K_pos_int)  "<K_pos_int>"
  Rate Transition8/1 -> Matrix Multiply1/2  "omega_dot_des"
  Initialized Output (with references)/1 -> Rate Transition/1, Bus Selector/1, Bus Selector9/1, Bus Assignment/1
  Bus Selector6/4 -> MATLAB Function1/7(K_acc)  "<K_acc>"
  Bus Selector6/3 -> MATLAB Function1/6(K_vel)  "<K_vel>"
  Bus Selector6/1 -> MATLAB Function1/4(K_pos)  "<K_pos>"
  External Inputs1/1 -> Rate Transition1/1
  Matrix Multiply1/1 -> Add2/2
  Add2/1 -> Reshape/1
  Bus Selector/1 -> Add/1  "<T>"
  Bus Selector3/3 -> MATLAB Function1/10(ai)  "<a_e>"
  Bus Selector3/2 -> MATLAB Function1/9(vi)  "<v_e>"
  Bus Selector3/4 -> MATLAB Function1/11(q)  "<q>"
  Bus Selector3/1 -> MATLAB Function1/8(pi)  "<p_e>"
  States/1 -> Rate Transition2/1
  Bus Selector5/3 -> MATLAB Function1/3(a_ref)  "<a>"
  Bus Selector5/2 -> MATLAB Function1/2(v_ref)  "<v>"
  Bus Selector5/1 -> MATLAB Function1/1(p_ref)  "<p>"
  Bus Assignment/1 -> Control System Outputs/1
  Reshape/1 -> Bus Assignment/3  "Tau"
  Add/1 -> Bus Assignment/2  "T"
  Bus Selector2/1 -> Product/2  "<m>"
  MATLAB Function1/1(T_des) -> Rate Transition3/1
  Bus Selector1/1 -> MATLAB Function2/6(q)  "<q>"
  Bus Selector1/2 -> MATLAB Function2/7(omega)  "<omega>"
  Bus Selector4/1 -> MATLAB Function2/2(q_ref)  "<q>"
  Bus Selector4/2 -> MATLAB Function2/3(omega_ref)  "<omega>"
  External Inputs/1 -> Bus Selector2/1, Rate Transition6/1
  Rate Transition7/1 -> Bus Selector1/1
  Bus Selector7/1 -> MATLAB Function2/4(K_att)  "<K_att>"
  Bus Selector7/2 -> MATLAB Function2/5(K_omega)  "<K_omega>"
  Rate Transition/1 -> Bus Selector5/1
  Rate Transition1/1 -> Bus Selector6/1
  Rate Transition2/1 -> Subsystem/1(States), Bus Selector3/1
  Product/1 -> Add/2
  MATLAB Function1/2(att_dir_correction_from_pos_) -> Rate Transition4/1  "omega_dot_des"
  Rate Transition4/1 -> MATLAB Function2/1(att_dir_correction_from_pos)
  Rate Transition3/1 -> Product/1
  Rate Transition6/1 -> Bus Selector7/1
  States1/1 -> Rate Transition7/1
  MATLAB Function2/1(omega_dot_des) -> Rate Transition8/1
  Rate Transition9/1 -> Bus Selector4/1
  Initialized Output (with references)1/1 -> Rate Transition9/1
  External Inputs2/1 -> Bus Selector8/1
  Bus Selector8/1 -> Matrix Multiply1/1  "<J>"
